simulink model "BMS_V4"  (R2017b)
settings: Solver=FixedStepDiscrete  StartTime=0.0  StopTime=inf  FixedStep=BASETIME  RelTol=1e-3  EnableMultiTasking=on
values from neighbouring files (symbols this model uses):
  AKT_BALANCE = uint16(8)    [BMS_V4_config.m]
  BALANCE = uint16(4)    [BMS_V4_config.m]
  BALANCE_RESISTOR = int32(5)    [BMS_V4_config.m]
  BALANCE_VEC = uint16(8)    [BMS_V4_config.m]
  CELL_SOC = uint16(7)    [BMS_V4_config.m]
  CELL_STATE = uint16(3)    [BMS_V4_config.m]
  CELL_TEMPERATURE = uint16(6)    [BMS_V4_config.m]
  CELL_VOLTAGE = uint16(5)    [BMS_V4_config.m]
  CELLACTBITFIELD = hex2dec('300')    [BMS_V4_config.m]
  CELLDEACTBITFIELD = hex2dec('100')    [BMS_V4_config.m]
  CELLT_BURST = uint16(6)    [BMS_V4_config.m]
  CELLV_BURST = uint16(5)    [BMS_V4_config.m]
  CLK_CYC_timer_1 = 586    [BMS_V4_config.m]
  CLK_CYC_timer_2 = 5860    [BMS_V4_config.m]
  CLK_CYC_timer_3 = 280    [BMS_V4_config.m]
  CLK_CYC_timer_4 = 586*100    (= 58600)    [BMS_V4_config.m]
  CLK_CYC_timer_5 = 5800*2    (= 11600)    [BMS_V4_config.m]
  CLK_CYC_timer_6 = 320    [BMS_V4_config.m]
  CN_CELLS = int32(40*3600)    [BMS_V4_config.m]
  CONTACTOR = uint16(1)    [BMS_V4_config.m]
  CONTACTOR_LOCKED = uint16(0)    [BMS_V4_config.m]
  CONTACTOR_UNLOCKED = uint16(1)    [BMS_V4_config.m]
  DEBUG_SEND_STATES = uint16(hex2dec('01'))    [BMS_V4_config.m]
  DELTA_SOC_BALANCE = int32(5*1e6)    [BMS_V4_config.m]
  DELTA_SOC_BALANCE_OFF = int32(1*1e5)    [BMS_V4_config.m]
  DETERMINE_MODEL_PARAMETER_ACT = uint16(100)    [BMS_V4_config.m]
  DETERMINE_MODEL_PARAMETER_SCC = uint16(101)    [BMS_V4_config.m]
  ERROR = uint16(1)    [BMS_V4_config.m]
  EXTERN_SIGNALS = uint16(1)    [BMS_V4_config.m]
  FREQUENCY_STEPS = uint16([25 50 75 100 150 250 500 750                                      1000 1500 2500 5000 7500                                      10010 10015 10025 10050 10075                                      10100 10150 10250 10500 10750                                      11000 11500])    [BMS_V4_config.m]
  GET_IMAG_PART_MFC = uint16(9)    [BMS_V4_config.m]
  GET_IMAG_PART_MSF = uint16(4)    [BMS_V4_config.m]
  GET_REAL_PART_MFC = uint16(8)    [BMS_V4_config.m]
  GET_REAL_PART_MSF = uint16(3)    [BMS_V4_config.m]
  IMU = uint16(7)    [BMS_V4_config.m]
  IMU_AMP_OFF = uint16(5)    [BMS_V4_config.m]
  IMU_DATA_READ_LOCUS_ACT = uint16(6)    [BMS_V4_config.m]
  IMU_DATA_READ_LOCUS_SCC = uint16(7)    [BMS_V4_config.m]
  IMU_DEBUG = uint16(9)    [BMS_V4_config.m]
  IMU_GET_DATA_MFC = uint16(8)    [BMS_V4_config.m]
  IMU_GET_DATA_MSF = uint16(3)    [BMS_V4_config.m]
  IMU_OFFSET_POLLING = uint16(11)    [BMS_V4_config.m]
  IMU_POLLING = uint16(2)    [BMS_V4_config.m]
  IMU_POWER = uint16(10)    [BMS_V4_config.m]
  IMU_SEND_IMAG = uint16(11)    [BMS_V4_config.m]
  IMU_SEND_REAL = uint16(10)    [BMS_V4_config.m]
  INDEX_IMAGPART = uint16(2)    [BMS_V4_config.m]
  INDEX_REALPART = uint16(1)    [BMS_V4_config.m]
  INFO = uint16(2)    [BMS_V4_config.m]
  INIT_OFFSET_AMPLITUDE = uint16(2)    [BMS_V4_config.m]
  LINE_CURRENT = uint16(3)    [BMS_V4_config.m]
  LINE_CURRENT_CANA = uint16(4)    [BMS_V4_config.m]
  LINE_CURRENT_SWITCH_THRESHOLD = int32(2*1e6)    [BMS_V4_config.m]
  NUM_OF_CELLS = uint16(16)    [BMS_V4_config.m]
  NUM_OF_FREQUENCIES_PSO = uint16(14)    [BMS_V4_config.m]
  NUM_OF_LINES = uint16(1)    [BMS_V4_config.m]
  NUM_OF_PARAMETER = single(5)    [BMS_V4_config.m]
  NUM_OF_SOC_POINTS = uint16(110)    [BMS_V4_config.m]
  P_L_BOUND = single([0.05;0.01;0.1;0.01;0.1])    [BMS_V4_config.m]
  P_U_BOUND = single([0.50;0.20;0.9;0.06;60])    [BMS_V4_config.m]
  PARA_ACT_SEND = uint16(101)    [BMS_V4_config.m]
  PARA_DATA_STORE_ACT = uint16(8)    [BMS_V4_config.m]
  PARA_DATA_STORE_SCC = uint16(9)    [BMS_V4_config.m]
  PARA_SCC_SEND = uint16(102)    [BMS_V4_config.m]
  PARTICLE_INIT = single(create_startparticle(P_L_BOUND,P_U_BOUND,NUM_OF_PARTICLE))    [BMS_V4_config.m]
  POLACT = hex2dec('00000BFF')    [BMS_V4_config.m]
  POLDEACT = hex2dec('000008FF')    [BMS_V4_config.m]
  PSO_PARA_DEBUG = uint16(13)    [BMS_V4_config.m]
  REQUEST_SOC_REF = uint16(1000)    [BMS_V4_config.m]
  SCALE_FACTOR_CH1 = single(0.66666666)    [BMS_V4_config.m]
  SCALE_FACTOR_CH2 = single(0.66666666)    [BMS_V4_config.m]
  SEND_CELL_SOC_ABS = uint16(199)    [BMS_V4_config.m]
  SHUT_DOWN_BALANCE_OFF = uint16(3)    [BMS_V4_config.m]
  SHUT_DOWN_BALANCE_ON = uint16(2)    [BMS_V4_config.m]
  START_IMU_MSL = uint16(3)    [BMS_V4_config.m]
  START_IMU_SCC = uint16(1)    [BMS_V4_config.m]
  SWITCH_IMU_OFF = uint16(2)    [BMS_V4_config.m]
  SWITCH_IMU_ON = uint16(1)    [BMS_V4_config.m]
  SWITCH_IMU_ON_OFF = uint16(4)    [BMS_V4_config.m]
  SYSTEM_DEBUG = uint16(12)    [BMS_V4_config.m]
  TIMEOUT_CANA = uint32(5000)    [BMS_V4_config.m]
  TIMEOUT_GATEWAY = uint32(500)    [BMS_V4_config.m]
  TS_SOC = single(0.010)    [BMS_V4_config.m]
  WARNING = uint16(2)    [BMS_V4_config.m]
libraries: c280xlib x44, c2833xlib x5, simulink x2, c2000lib x1, idelinklib_common x1
(part 8 of 8)

== stateflow chart BMS_V4/Chart ==
  state init
    en:
  state user_read_imu_data_scc
    state get_imu_data_soc_scc_from_mram
      en:
      soc_point_send_CANA  = uint16(1);
      freq_point_send_CANA = uint16(0);
      cellNo_read = user_request_cellno_CANA;
      mram_command[SOC_SCC_READ - uint16(1)] = true;
    state get_imu_data_locus_scc_from_mram
      en:
      freq_point_send_CANA = uint16(0);
      mram_cellno_to_read = cellNo_read;
      mram_soc_point_to_read = soc_point_send_CANA;
      mram_command[IMU_DATA_READ_LOCUS_SCC - uint16(1)] = true;
    state get_imu_data_locus_scc_from_mram1
      en:
      soc_point_send_CANA = user_request_socpoint_CANA;
      freq_point_send_CANA = uint16(0);
      mram_cellno_to_read = cellNo_read;
      mram_soc_point_to_read = soc_point_send_CANA;
      mram_command[IMU_DATA_READ_LOCUS_SCC - uint16(1)] = true;
    state send_can_cell_imu_real_part
      en:
      [imu_debug_CAN_low,imu_debug_CAN_high]=IMU_debug_send_cell_real(cellNo_read, ...
      freq_point_send_CANA+uint16(1),...
      soc_points_of_scc[soc_point_send_CANA- uint16(1)],...
      one_locus_scc[freq_point_send_CANA][uint16(0)]);
      CANA_send_data[IMU_SEND_REAL - uint16(1)] = true;
    state send_can_cell_imu_imag_part
      en:
      [imu_debug_CAN_low,imu_debug_CAN_high]=IMU_debug_send_cell_imag(cellNo_read, ...
      freq_point_send_CANA+uint16(1),...
      soc_points_of_scc[soc_point_send_CANA- uint16(1)],...
      one_locus_scc[freq_point_send_CANA][uint16(1)]);
      CANA_send_data[IMU_SEND_IMAG - uint16(1)] = true;
    get_imu_data_soc_scc_from_mram -> (junction 69) : [mram_command[SOC_SCC_READ - uint16(1)] == false]
    (junction 69) -> get_imu_data_locus_scc_from_mram1 [order 2]
    (junction 69) -> get_imu_data_locus_scc_from_mram [order 1] : [user_request_socpoint_CANA < uint16(1)]
    (junction 80) -> get_imu_data_locus_scc_from_mram [order 1] : //[soc_point_send_CANA < NUM_OF_SOC_POINTS]
        | [(soc_point_send_CANA < last_soc_point_index) && (user_request_socpoint_CANA < uint16(1))]
        | {soc_point_send_CANA++;}
    (junction 72) -> (junction 80) [order 2]
    get_imu_data_locus_scc_from_mram -> user_read_imu_data_scc.send_can_cell_imu_real_part : [mram_command[IMU_DATA_READ_LOCUS_SCC - uint16(1)] == false]
    get_imu_data_locus_scc_from_mram1 -> user_read_imu_data_scc.send_can_cell_imu_real_part : [mram_command[IMU_DATA_READ_LOCUS_SCC - uint16(1)] == false]
    (junction 72) -> user_read_imu_data_scc.send_can_cell_imu_real_part [order 1] : [freq_point_send_CANA < NUM_OF_FREQUENCIES]
    (junction 70) -> (junction 72)
    user_read_imu_data_scc.send_can_cell_imu_real_part -> user_read_imu_data_scc.send_can_cell_imu_imag_part : //after(TIMER_IMU_DEBUG_SEND_DATA,sec)
        | [CANA_send_data[IMU_SEND_REAL - uint16(1)] == false]
    user_read_imu_data_scc.send_can_cell_imu_imag_part -> (junction 70) : //after(TIMER_IMU_DEBUG_SEND_DATA,sec)
        | [CANA_send_data[IMU_SEND_IMAG - uint16(1)] == false]
        | {freq_point_send_CANA++;}
  state user_read_imu_data_act
    state get_imu_data_act_from_mram
      en:
      cellNo_read  = uint16(1);
      freq_point_send_CANA = uint16(0);
    state get_imu_data_locus_act_from_mram_all_cells
      en:
      freq_point_send_CANA = uint16(0);
      mram_cellno_to_read = cellNo_read;
      mram_command[IMU_DATA_READ_LOCUS_ACT - uint16(1)] = true;
    state get_imu_data_locus_act_from_mram_one_cell
      en:
      cellNo_read = user_request_cellno_CANA;
      freq_point_send_CANA = uint16(0);
      mram_cellno_to_read = cellNo_read;
      mram_command[IMU_DATA_READ_LOCUS_ACT - uint16(1)] = true;
    state send_can_cell_imu_real_part
      en:
      [imu_debug_CAN_low,imu_debug_CAN_high]=IMU_debug_send_cell_real(cellNo_read, ...
      freq_point_send_CANA+uint16(1),...
      soc_of_one_locus_act,...
      one_locus_act[freq_point_send_CANA][uint16(0)]);
      CANA_send_data[IMU_SEND_REAL - uint16(1)] = true;
    state send_can_cell_imu_imag_part
      en:
      [imu_debug_CAN_low,imu_debug_CAN_high]=IMU_debug_send_cell_imag(cellNo_read, ...
      freq_point_send_CANA+uint16(1),...
      soc_of_one_locus_act,...
      one_locus_act[freq_point_send_CANA][uint16(1)]);
      CANA_send_data[IMU_SEND_IMAG - uint16(1)] = true;
    get_imu_data_act_from_mram -> (junction 105)
    (junction 105) -> get_imu_data_locus_act_from_mram_one_cell [order 2]
    (junction 105) -> get_imu_data_locus_act_from_mram_all_cells [order 1] : [user_request_cellno_CANA < uint16(1)]
    (junction 106) -> get_imu_data_locus_act_from_mram_all_cells [order 1] : //[soc_point_send_CANA < NUM_OF_SOC_POINTS]
        | [(cellNo_read < NUM_OF_CELLS) && (user_request_cellno_CANA < uint16(1))]
        | {cellNo_read++;}
    (junction 107) -> (junction 106) [order 2]
    get_imu_data_locus_act_from_mram_all_cells -> user_read_imu_data_act.send_can_cell_imu_real_part : [mram_command[IMU_DATA_READ_LOCUS_ACT - uint16(1)] == false]
    get_imu_data_locus_act_from_mram_one_cell -> user_read_imu_data_act.send_can_cell_imu_real_part : [mram_command[IMU_DATA_READ_LOCUS_ACT - uint16(1)] == false]
    (junction 107) -> user_read_imu_data_act.send_can_cell_imu_real_part [order 1] : [freq_point_send_CANA < NUM_OF_FREQUENCIES]
    (junction 108) -> (junction 107)
    user_read_imu_data_act.send_can_cell_imu_real_part -> user_read_imu_data_act.send_can_cell_imu_imag_part : //after(TIMER_IMU_DEBUG_SEND_DATA,sec)
        | [CANA_send_data[IMU_SEND_REAL - uint16(1)] == false]
    user_read_imu_data_act.send_can_cell_imu_imag_part -> (junction 108) : //after(TIMER_IMU_DEBUG_SEND_DATA,sec)
        | [CANA_send_data[IMU_SEND_IMAG - uint16(1)] == false]
        | {freq_point_send_CANA++;}
  state user_read_para_data_scc
    state init
      en:
      cellNo_read = uint16(1);
    state get_para_data_scc_all_cells
      en:
      para_act_cellno = cellNo_read;
      mram_command[PARA_DATA_READ_SCC-uint16(1)] =true;
    state get_para_data_scc_one_cell
      en:
      cellNo_read = user_request_cellno_CANA;
      para_act_cellno = cellNo_read;
      mram_command[PARA_DATA_READ_SCC-uint16(1)] =true;
    state send_can_para_data_scc
      en:
      para_send_act_cell_CANA = cellNo_read;
      para_send_act_or_scc_CANA = PARA_SCC_SEND;
      CANA_send_data[PSO_PARA_DEBUG-uint16(1)]=true;
    user_read_para_data_scc.init -> (junction 141)
    (junction 141) -> get_para_data_scc_one_cell [order 2]
    (junction 141) -> user_read_para_data_scc.get_para_data_scc_all_cells [order 1] : [user_request_cellno_CANA < uint16(1)]
    (junction 142) -> user_read_para_data_scc.get_para_data_scc_all_cells [order 1] : //[soc_point_send_CANA < NUM_OF_SOC_POINTS]
        | [(cellNo_read < NUM_OF_CELLS) && (user_request_cellno_CANA < uint16(1))]
        | {cellNo_read++;}
    (junction 143) -> (junction 142)
    user_read_para_data_scc.get_para_data_scc_all_cells -> user_read_para_data_scc.send_can_para_data_scc : [mram_command[PARA_DATA_READ_SCC - uint16(1)] == false]
    get_para_data_scc_one_cell -> user_read_para_data_scc.send_can_para_data_scc : [mram_command[PARA_DATA_READ_SCC - uint16(1)] == false]
    user_read_para_data_scc.send_can_para_data_scc -> (junction 143) : [CANA_send_data[PSO_PARA_DEBUG-uint16(1)] == false]
  state user_read_para_data_act
    state init
      en:
      cellNo_read = uint16(1);
    state get_para_data_scc_all_cells
      en:
      para_act_cellno = cellNo_read;
      mram_command[PARA_DATA_READ_ACT-uint16(1)] =true;
    state send_can_para_data_scc
      en:
      para_send_act_cell_CANA = cellNo_read;
      para_send_act_or_scc_CANA = PARA_ACT_SEND;
      CANA_send_data[PSO_PARA_DEBUG-uint16(1)]=true;
    user_read_para_data_act.init -> user_read_para_data_act.get_para_data_scc_all_cells
    (junction 183) -> user_read_para_data_act.get_para_data_scc_all_cells [order 1] : //[soc_point_send_CANA < NUM_OF_SOC_POINTS]
        | [cellNo_read < NUM_OF_CELLS ]
        | {cellNo_read++;}
    (junction 184) -> (junction 183)
    user_read_para_data_act.get_para_data_scc_all_cells -> user_read_para_data_act.send_can_para_data_scc : [mram_command[PARA_DATA_READ_SCC - uint16(1)] == false]
    user_read_para_data_act.send_can_para_data_scc -> (junction 184) : [CANA_send_data[PSO_PARA_DEBUG-uint16(1)] == false]
  (junction 106) -> (junction 132) [order 2] : {user_interface[USER_READ_ACT_FOR_CELLNO - uint16(1)] = false;}
  (junction 200) -> user_read_para_data_act.init : [user_interface[USER_READ_PARA_ACT_FOR_CELLNO-uint16(1)] == true]
  (junction 166) -> user_read_para_data_scc.init [order 1] : [user_interface[USER_READ_PARA_SCC_FOR_CELLNO-uint16(1)] == true]
  (junction 128) -> get_imu_data_act_from_mram [order 1] : [user_interface[USER_READ_ACT_FOR_CELLNO-uint16(1)] == true]
  (junction 91) -> get_imu_data_soc_scc_from_mram [order 1] : [user_interface[USER_READ_SCC_FOR_CELLNO-uint16(1)] == true]
  (junction 142) -> (junction 164) [order 2] : {user_interface[USER_READ_PARA_SCC_FOR_CELLNO - uint16(1)] = false;}
  (junction 183) -> (junction 204) [order 2] : {user_interface[USER_READ_PARA_ACT_FOR_CELLNO - uint16(1)] = false;}
  (default) -> init
  init -> (junction 98) : [ (user_interface[0] || ...
      |    user_interface[1] || ...
      |    user_interface[2] || ...
      |    user_interface[3] || ...
      |    user_interface[4] || ...
      |    user_interface[5] || ...
      |    user_interface[6] || ...
      |    user_interface[7] || ...
      |    user_interface[8] || ...
      |    user_interface[9] ) != 0]
  (junction 98) -> (junction 91)
  (junction 96) -> init
  (junction 132) -> (junction 96)
  (junction 91) -> (junction 128) [order 2]
  (junction 80) -> (junction 96) [order 2] : {user_interface[USER_READ_SCC_FOR_CELLNO - uint16(1)] = false;}
  (junction 164) -> (junction 132)
  (junction 128) -> (junction 166) [order 2]
  (junction 204) -> (junction 164)
  (junction 166) -> (junction 200) [order 2]
  data: cellNo function_input uint16; freq_id function_input uint16; soc function_input int32; cell_real_part function_input single; CAN_LOW function_output uint32; CAN_HIGH function_output uint32; cellNo function_input uint16; freq_id function_input uint16; soc function_input int32; cell_imag_part function_input single; CAN_LOW function_output uint32; CAN_HIGH function_output uint32; user_request_cellno_CANA data_store_memory; soc_point_send_CANA local uint16; freq_point_send_CANA local uint16; cellNo_read local uint16; mram_command data_store_memory; IMU_DATA_READ_LOCUS_SCC parameter; one_locus_scc data_store_memory; imu_debug_CAN_low data_store_memory; imu_debug_CAN_high data_store_memory; CANA_send_data data_store_memory; IMU_SEND_REAL parameter; IMU_SEND_IMAG parameter; TIMER_IMU_DEBUG_SEND_DATA parameter; NUM_OF_FREQUENCIES parameter; SOC_SCC_READ parameter; soc_points_of_scc data_store_memory; NUM_OF_SOC_POINTS parameter; USER_READ_SCC_FOR_CELLNO parameter; user_interface data_store_memory; mram_cellno_to_read data_store_memory; mram_soc_point_to_read data_store_memory; FREQUENCY_STEPS parameter; last_soc_point_index data_store_memory; user_request_socpoint_CANA data_store_memory; USER_READ_ACT_FOR_CELLNO parameter; one_locus_act data_store_memory; soc_of_one_locus_act data_store_memory; IMU_DATA_READ_LOCUS_ACT parameter; NUM_OF_CELLS parameter; para_act_cellno data_store_memory; para_send_act_cell_CANA data_store_memory; para_send_act_or_scc_CANA data_store_memory; PARA_DATA_READ_SCC parameter; PARA_SCC_SEND parameter; PSO_PARA_DEBUG parameter; USER_READ_PARA_SCC_FOR_CELLNO parameter; PARA_ACT_SEND parameter; PARA_DATA_READ_ACT parameter; USER_READ_PARA_ACT_FOR_CELLNO parameter
  events: trigger_user_interface input FUNCTION_CALL_EVENT
  function [CAN_LOW, CAN_HIGH] = IMU_debug_send_cell_real(cellNo,freq_id,soc,cell_real_part):
    | function [CAN_LOW, CAN_HIGH] = IMU_debug_send_cell_real(cellNo,freq_id,soc,cell_real_part)
    |  
    | CODE = uint16([0 0 0 0 0 0 0 0]);
    | 
    | soc_s=single(soc);
    | soc_convert = typecast(soc/1e6,'uint32');  
    | soc1 = uint16(bitand(uint32(hex2dec('000000FF')),soc_convert));
    | frequence=FREQUENCY_STEPS(freq_id);
    | real_part=typecast(cell_real_part,'uint32');
    | 
    | CODE(1)= uint16(bitand(uint16(hex2dec('00ff')),uint16(cellNo)));
    | CODE(2)= uint16(bitand(uint16(hex2dec('00ff')),uint16(frequence)));
    | CODE(3)= uint16(bitand(uint16(hex2dec('00ff')),bitshift(uint16(frequence),-8)));
    | CODE(4)= uint16(bitand(uint16(hex2dec('00ff')),uint16(soc1)));
    | 
    | CODE(5)= uint16(bitand(uint32(hex2dec('000000ff')),real_part));
    | CODE(6)= uint16(bitand(uint32(hex2dec('000000ff')),bitshift(real_part,-8)));
    | CODE(7)= uint16(bitand(uint32(hex2dec('000000ff')),bitshift(real_part,-16)));
    | CODE(8)= uint16(bitand(uint32(hex2dec('000000ff')),bitshift(real_part,-24)));
    | 
    | x1=uint16(bitand(uint16(hex2dec('00ff')),uint16(CODE(1))));
    | x2=uint16(bitand(uint16(hex2dec('ff00')),uint16(bitshift(uint16(CODE(2)),8))));
    | x3=uint16(bitand(uint16(hex2dec('00ff')),uint16(CODE(3))));
    | x4=uint16(bitand(uint16(hex2dec('ff00')),uint16(bitshift(uint16(CODE(4)),8))));
    | 
    | x11=uint16(bitor(x1,x2));
    | x12=uint16(bitor(x3,x4));
    | 
    | out1=uint32(bitor(uint32(x11),bitshift(uint32(x12),16)));
    | 
    | x5=uint16(bitand(uint16(hex2dec('00ff')),uint16(CODE(5))));
    | x6=uint16(bitand(uint16(hex2dec('ff00')),uint16(bitshift(uint16(CODE(6)),8))));
    | x7=uint16(bitand(uint16(hex2dec('00ff')),uint16(CODE(7))));
    | x8=uint16(bitand(uint16(hex2dec('ff00')),uint16(bitshift(uint16(CODE(8)),8))));
    | 
    | x21=uint16(bitor(x5,x6));
    | x22=uint16(bitor(x7,x8));
    | 
    | out2=uint32(bitor(uint32(x21),bitshift(uint32(x22),16)));
    | 
    | CAN_LOW=out1;
    | CAN_HIGH=out2;
  function [CAN_LOW, CAN_HIGH] = IMU_debug_send_cell_imag(cellNo,freq_id,soc,cell_imag_part):
    | function [CAN_LOW, CAN_HIGH] = IMU_debug_send_cell_imag(cellNo,freq_id,soc,cell_imag_part)
    |  
    | CODE = uint16([0 0 0 0 0 0 0 0]);
    | 
    | soc_s=single(soc);
    | soc_convert = typecast(soc/1e6,'uint32');  
    | soc1 = uint16(bitand(uint32(hex2dec('000000FF')),soc_convert));
    | frequence=FREQUENCY_STEPS(freq_id);
    | imag_part=typecast(cell_imag_part,'uint32');
    | 
    | CODE(1)= uint16(bitand(uint16(hex2dec('00ff')),uint16(cellNo)));
    | CODE(2)= uint16(bitand(uint16(hex2dec('00ff')),uint16(frequence)));
    | CODE(3)= uint16(bitand(uint16(hex2dec('00ff')),bitshift(uint16(frequence),-8)));
    | CODE(4)= uint16(bitand(uint16(hex2dec('00ff')),uint16(soc1)));
    | 
    | CODE(5)= uint16(bitand(uint32(hex2dec('000000ff')),imag_part));
    | CODE(6)= uint16(bitand(uint32(hex2dec('000000ff')),bitshift(imag_part,-8)));
    | CODE(7)= uint16(bitand(uint32(hex2dec('000000ff')),bitshift(imag_part,-16)));
    | CODE(8)= uint16(bitand(uint32(hex2dec('000000ff')),bitshift(imag_part,-24)));
    | 
    | x1=uint16(bitand(uint16(hex2dec('00ff')),uint16(CODE(1))));
    | x2=uint16(bitand(uint16(hex2dec('ff00')),uint16(bitshift(uint16(CODE(2)),8))));
    | x3=uint16(bitand(uint16(hex2dec('00ff')),uint16(CODE(3))));
    | x4=uint16(bitand(uint16(hex2dec('ff00')),uint16(bitshift(uint16(CODE(4)),8))));
    | 
    | x11=uint16(bitor(x1,x2));
    | x12=uint16(bitor(x3,x4));
    | 
    | out1=uint32(bitor(uint32(x11),bitshift(uint32(x12),16)));
    | 
    | x5=uint16(bitand(uint16(hex2dec('00ff')),uint16(CODE(5))));
    | x6=uint16(bitand(uint16(hex2dec('ff00')),uint16(bitshift(uint16(CODE(6)),8))));
    | x7=uint16(bitand(uint16(hex2dec('00ff')),uint16(CODE(7))));
    | x8=uint16(bitand(uint16(hex2dec('ff00')),uint16(bitshift(uint16(CODE(8)),8))));
    | 
    | x21=uint16(bitor(x5,x6));
    | x22=uint16(bitor(x7,x8));
    | 
    | out2=uint32(bitor(uint32(x21),bitshift(uint32(x22),16)));
    | 
    | CAN_LOW=out1;
    | CAN_HIGH=out2;

== matlab function BMS_V4/FunctionCall_CANB_RX/handle_line_current/line_current_proceeding_KLARIC ==
  data: msg input; line_currents data_store_memory
function line_current_proceedng_KLARIC(msg)

global line_currents;
line_no = uint16(1);

%check sign



sign = uint16(bitand(uint32(hex2dec('00000001')),...
    bitshift(msg(1),-23)));

if (sign > uint16(0)) % negativ current
    current_u = uint32(bitor (uint32(hex2dec('FF000000')),...
        bitand(uint32(hex2dec('00FFFFFF')),msg(1))));
else % positive current
    current_u = uint32(bitand(uint32(hex2dec('00FFFFFF')),msg(1)));
end

current = typecast(current_u,'int32'); %current mA
current = current*1e3; % current µA

line_currents(line_no)=current;

== matlab function BMS_V4/FunctionCall_CANA_RX/handle_line_current/line_current_proceeding ==
  data: msg input; next_gateway_request data_store_memory; current_CH1 output; current_CH2 output; line_no output; activate_current_correction data_store_memory; correction_current_CH1 data_store_memory; correction_current_CH2 data_store_memory
function [current_CH1, current_CH2,line_no]=line_current_proceedng(msg)

global activate_current_correction;
global correction_current_CH1;
global correction_current_CH2;


line_no = uint16(bitand(uint32(hex2dec('000000FF')),msg(1)))+uint16(1);

current_V_CH1 = uint16(bitand(uint32(hex2dec('0000FFFF')),...
    bitshift(msg(1),-8)));

current_V_CH2 = uint16(bitor(bitand(uint32(hex2dec('000000FF')),...
    bitshift(msg(1),-24)),bitand(uint32(hex2dec('0000FF00')),...
    bitshift(msg(2),8))));

if(activate_current_correction == true)
    
    correction_current_CH1 = single(current_V_CH1)/single(1e4);
    correction_current_CH2 = single(current_V_CH2)/single(1e4);
    activate_current_correction = false;
    
end

current_CH1 = current_V_CH1;
current_CH2 = current_V_CH2;

== matlab function BMS_V4/FunctionCall_CANA_RX/handle_line_current/line_current_proceeding_KLARIC ==
  data: msg input; line_currents data_store_memory
function line_current_proceedng_KLARIC(msg)

global line_currents;
line_no = uint16(1);

%check sign



sign = uint16(bitand(uint32(hex2dec('00000001')),...
    bitshift(msg(1),-23)));

if (sign > uint16(0)) % negativ current
    current_u = uint32(bitor (uint32(hex2dec('FF000000')),...
        bitand(uint32(hex2dec('00FFFFFF')),msg(1))));
else % positive current
    current_u = uint32(bitand(uint32(hex2dec('00FFFFFF')),msg(1)));
end

current = typecast(current_u,'int32'); %current mA
current = current*1e3; % current µA

line_currents(line_no)=current;

== matlab function BMS_V4/FunctionCall_CANA_RX/handle_line_current/save_current ==
  data: current input; line_no input; next_gateway_request data_store_memory; line_currents data_store_memory; LINE_CURRENT parameter; gateway_request data_store_memory
function save_current(current,line_no, LINE_CURRENT)
% Datenempfang über CAN

global line_currents;
global next_gateway_request;
global gateway_request;

line_currents(line_no)=current;
%line_currents(line_no)=int32(0);

gateway_request(LINE_CURRENT) = false;
next_gateway_request = true;

== matlab function BMS_V4/FunctionCall_CANB_RX/handle_active_balance/balance_proceeding ==
  data: msg input; next_gateway_request data_store_memory; gateway_request data_store_memory; BALANCE parameter; active_balance_vector data_store_memory; NUM_OF_CELLS parameter
function balance_proceedng(msg, BALANCE, NUM_OF_CELLS)

global next_gateway_request;
global gateway_request;

global active_balance_vector;


%cell Number 1 to 16 => cells 

%cell Number 255 => no cell activ while polling

Cellnum =   uint16(bitand(uint32(hex2dec('000000FF')),bitshift(msg(1),-0)));
BatStat =   uint16(bitand(uint32(hex2dec('00000001')),bitshift(msg(1),-8)));
CellStat =  uint16(bitand(uint32(hex2dec('00000001')),bitshift(msg(1),-9)));
CellFull =  uint16(bitand(uint32(hex2dec('00000001')),bitshift(msg(1),-10)));
Polling =   uint16(bitand(uint32(hex2dec('00000001')),bitshift(msg(1),-11)));
%Notused = uint16(bitand(uint32(hex2dec('0000000F')),bitshift(msg(1),-12)));
actualCurrent = uint16(bitand(uint32(hex2dec('000000FF')),bitshift(msg(1),-16)));

actualCharge  = uint32(msg(2));

% if Polling >= 1 % Answer to polling
%     
%  if Cellnum > NUM_OF_CELLS % No Cell activ
%  
%      active_balance_vector(3,:)= 0;
%  else                         %Active cell
%  
%      active_balance_vector(3,Cellnum)= 1;
%      active_balance_vector(4,Cellnum)= actualCharge;
%      
%  end
%  
% else % Answer to Enable, disable or finish activ Balancing for Cell
%  
%  if Cellnum <= NUM_OF_CELLS
%   
%   if CellFull >= 1 %cell fully charged
%     %active_balance_vector(3,Cellnum)= 0; 
%   end
%     active_balance_vector(3,Cellnum)= 1;
%   % active_balance_vector(4,cellnum)= 0;
%   
%   
%  end  
%     
% end

if (Cellnum <= NUM_OF_CELLS)
  if CellStat > 0  
    active_balance_vector(3,Cellnum)= uint32(1);
    active_balance_vector(4,Cellnum)= actualCharge;
  else
    active_balance_vector(3,Cellnum)= uint32(0);
  end
elseif Cellnum > NUM_OF_CELLS
    
    active_balance_vector(3,:)= uint32(0);
    
end


%t.b.d
%code = uint16(bitand(uint32(hex2dec('000000FF')),msg(1)));

% gateway_request(BALANCE) = false;  
next_gateway_request=true;

== stateflow chart BMS_V4/Balancing ==
  state init
    en:
  state checking
    en:
    [bal_need,bal_on] = Check_SoC_balance()
  state can_activation [commented out]
    en:
    gateway_request(AKT_BALANCE-uint16(1)) = 1;
  (default) -> init
  init -> checking
  checking -> init
  checking -> can_activation [commented out] : [((balance_flag == 1)&&(bal_need == 1)) || ((balance_flag == 0)&&(bal_on == 1))]
  data: balance_need_out function_output uint32; balance_on_out function_output uint32; cell_soc_CC data_store_memory; DELTA_SOC_BALANCE parameter double; active_balance_vector data_store_memory; balance_flag data_store_memory; CN_CELLS parameter double; DELTA_SOC_BALANCE_OFF parameter double; gateway_request data_store_memory; bal_need local double; bal_on local double; AKT_BALANCE parameter
  events: trigger_activ_blancing input FUNCTION_CALL_EVENT
  function [balance_need_out, balance_on_out ]= Check_SoC_balance:
    | function [balance_need_out, balance_on_out ]= Check_SoC_balance
    | 
    | global cell_soc_CC
    | global active_balance_vector
    | 
    | 
    | balance_need = zeros(length(cell_soc_CC),1);
    | delta_SoC_need = int32(zeros(length(cell_soc_CC),1));
    | 
    | maxSoC= int32(max(cell_soc_CC(:,1)));
    | 
    |  for k = 1:1:length(cell_soc_CC)
    |     
    |    if maxSoC > (cell_soc_CC(k,1) + DELTA_SOC_BALANCE)
    |        
    |     balance_need(k,1)   = 1 ;
    |     delta_SoC_need(k,1) = maxSoC - cell_soc_CC(k,1);
    |        
    |    elseif maxSoC < (cell_soc_CC(k,1) + DELTA_SOC_BALANCE_OFF)
    |     
    |      balance_need(k,1)   = 0 ;
    |      delta_SoC_need(k,1) = 0 ;
    |      
    |    end
    |    
    |    
    |     
    |  end
    | 
    |  delta_charge_need = ((single(delta_SoC_need / 1e8)) * single(CN_CELLS / 3600) * 1000); % Convert SoC to mAh
    |  
    |  active_balance_vector(1:end,1) = balance_need;
    |  d_charge_need = typecast(delta_charge_need,'uint32');
    |  active_balance_vector(1:end,2) = uint32(d_charge_need);
    |  balance_need_out = uint32(max(balance_need));
    |  balance_on_out = max(active_balance_vector(:,3));
    |  
    | end
